simulink model "modelo_no_lineal"  (R2018a)
settings: Solver=VariableStepAuto  StartTime=0.0  StopTime=10.0  RelTol=1e-3
settings Model: SimulationMode=external  Creator=Guido L  LastModifiedBy=Guido L

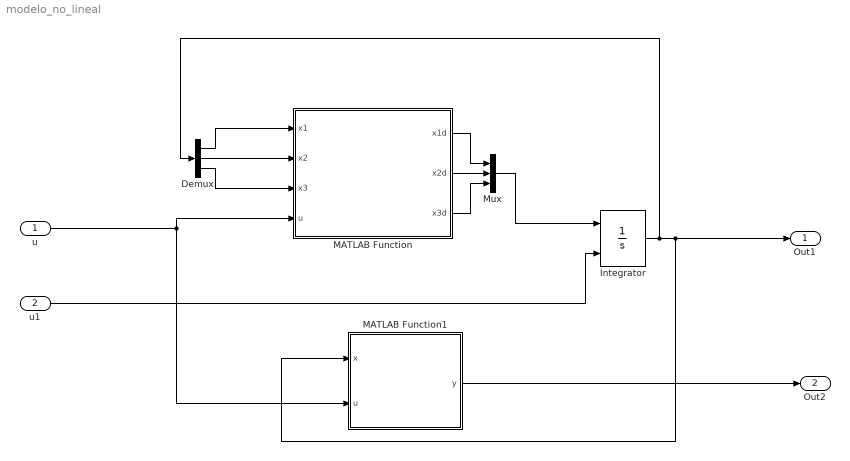
== system modelo_no_lineal ==
  u : Inport
  u1 : Inport  Port=2
  Demux : Demux  Outputs=3
  Integrator : Integrator  InitialConditionSource=external
  MATLAB Function : MATLAB Function  TreatAsAtomicUnit=on
  MATLAB Function1 : MATLAB Function  TreatAsAtomicUnit=on
  Mux : Mux  Inputs=3
  Out1 : Outport  SignalName=X
  Out2 : Outport  Port=2  SignalName=Y
  wires:
  MATLAB Function/1(x1d) -> Mux/1
  MATLAB Function/2(x2d) -> Mux/2
  MATLAB Function/3(x3d) -> Mux/3
  Mux/1 -> Integrator/1
  u1/1 -> Integrator/2
  Demux/1 -> MATLAB Function/1(x1)
  Demux/2 -> MATLAB Function/2(x2)
  Demux/3 -> MATLAB Function/3(x3)
  Integrator/1 -> Out1/1, MATLAB Function1/1(x), Demux/1
  MATLAB Function1/1(y) -> Out2/1
  u/1 -> MATLAB Function/4(u), MATLAB Function1/2(u)

== matlab function modelo_no_lineal/MATLAB Function1 ==
  data: x input; u input; y output
function y = fcn(x,u)
y = x(1);

== matlab function modelo_no_lineal/MATLAB Function ==
  data: x1 input; x2 input; x3 input; u input; x1d output; x2d output; x3d output
function [x1d, x2d, x3d] = fcn(x1, x2, x3, u)

    g=10;
    m=0.2;
    L=1;
    R=1;
    
    f1 = 0.5*(2+x3)^2/(1-x1)^2;
    f2 = 0.5*(2-x3)^2/(1+x1)^2;
        
    x1d = x2;
    x2d = -g + f1/m - f2/m;
    x3d = abs(x3)*x3*R/L+u/L;
